simulink model "plant_model"  (R2023b)
settings: Solver=VariableStepAuto  StartTime=0.0  StopTime=10.0  RelTol=1e-3
undefined symbols (not defined in the file or in its folder): K, K_theta, K_w, tau
settings Model: Creator=john  LastModifiedBy=john

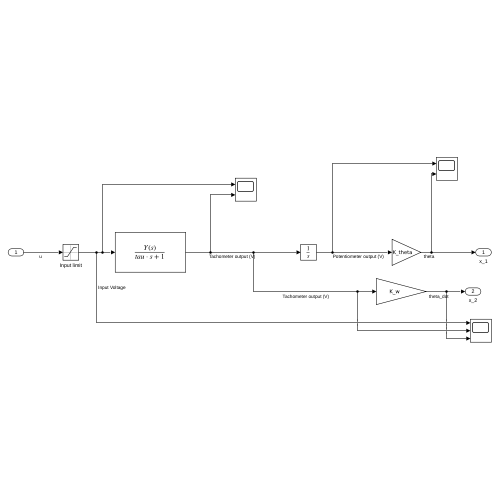
[thumbnail: Simulink's stored preview of the top-level diagram]
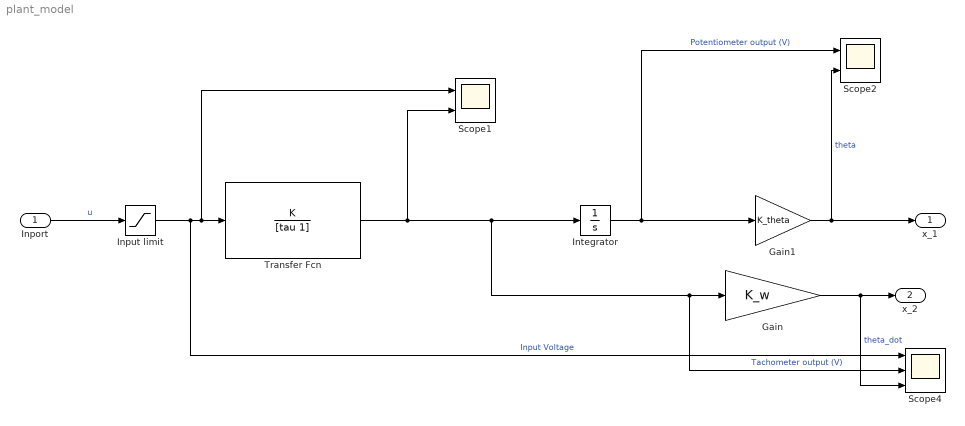
== system plant_model ==
  Inport : Inport
  Gain : Gain  Gain=K_w
  Gain1 : Gain  Gain=K_theta
  Input limit : Saturate  UpperLimit=5  LowerLimit=-5
  Integrator : Integrator
  Scope1 : Scope  NumInputPorts=2
  Scope2 : Scope  NumInputPorts=2
  Scope4 : Scope  NumInputPorts=3
  Transfer Fcn : TransferFcn  Numerator=K  Denominator=[tau 1]
  x_1 : Outport
  x_2 : Outport  Port=2
  wires:
  Inport/1 -> Input limit/1  "u"
  Integrator/1 -> Scope2/1, Gain1/1  "Potentiometer output (V)"
  Gain/1 -> Scope4/3, x_2/1  "theta_dot"
  Gain1/1 -> Scope2/2, x_1/1  "theta"
  Input limit/1 -> Scope4/1, Scope1/1, Transfer Fcn/1  "Input Voltage"
  Transfer Fcn/1 -> Scope1/2, Gain/1, Scope4/2, Integrator/1  "Tachometer output (V)"
